simulink model "CANTXcommunication"  (R2024a)
settings: Solver=VariableStepAuto  StartTime=0.0  StopTime=10.0  RelTol=1e-3
undefined symbols (not defined in the file or in its folder): canChannel
libraries: canlib x2, canmsglib x1
settings Model: DataDictionary=BMS_System_dict1.sldd  Creator=hirah  LastModifiedBy=hirah

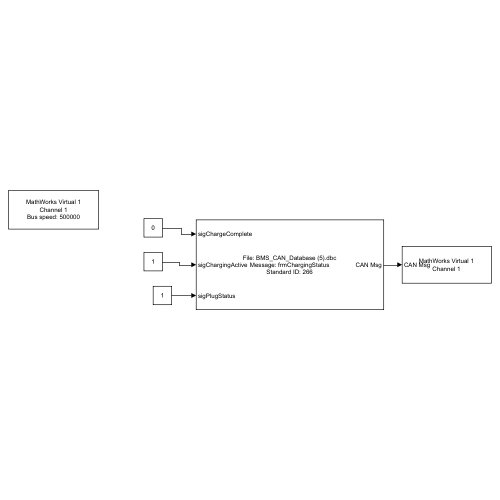
[thumbnail: Simulink's stored preview of the top-level diagram]
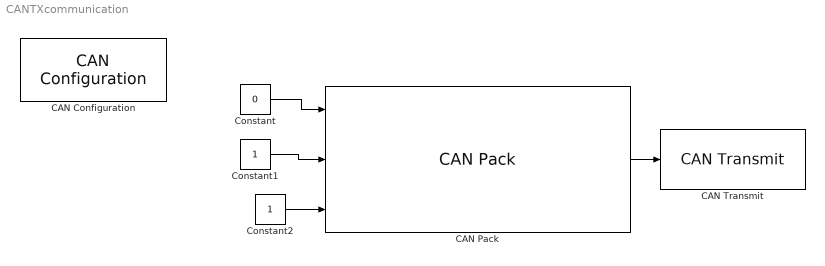
== system CANTXcommunication ==
  CAN Configuration : canlib/CAN Configuration  BlockHandle=708.0002  Device=MathWorks Virtual 1 (Channel 1)  DeviceMenu=MathWorks Virtual 1 (Channel 1)  ObjConstructor=canChannel('MathWorks', 'Virtual 1', 1)  BusSpeed=500000  EnableBitParameters=off  AckMode=Normal
  CAN Pack : canmsglib/CAN Pack  CANdbFile=C:\Users\hirah\Downloads\BMS_CAN_Database (5).dbc  MsgList=frmChargingStatus  MsgName=frmChargingStatus  MsgIDType=Standard (11-bit identifier)  MsgIdentifier=266  MsgLength=3  Remote=off  ApplyMinMax=off  BusOutput=off  SignalInfo={'sigChargeComplete','16','8','LE','unsigned','Standard','0','1','0','0','1';'sigChargingActive','8','8','LE','unsigned','Standard','0','1','0','0','1';'sigPlugStatus','0','8','LE','unsigned','Standard','0','1','0','0','2'}
      settings: LibrarySourceBlock=canlib/CAN Pack  DataFormat=CANdb specified signals
  CAN Transmit : canlib/CAN Transmit  BlockHandle=714.0001  Device=MathWorks Virtual 1 (Channel 1)  DeviceMenu=MathWorks Virtual 1 (Channel 1)  ObjConstructor=canChannel('MathWorks', 'Virtual 1', 1)  EnableEventTransmit=off  EnablePeriodicTransmit=off  MessagePeriod=1.000
  Constant : Constant  Value=0  OutDataTypeStr=uint8
  Constant1 : Constant  OutDataTypeStr=uint8
  Constant2 : Constant  OutDataTypeStr=uint8
  wires:
  CAN Pack/1 -> CAN Transmit/1
  Constant/1 -> CAN Pack/1
  Constant2/1 -> CAN Pack/3
  Constant1/1 -> CAN Pack/2
